simulink model "task2_2"  (R2023a)
settings: Solver=VariableStepAuto  StartTime=0.0  StopTime=10.0  RelTol=1e-3
settings Model: Creator=vasil  LastModifiedBy=vasil

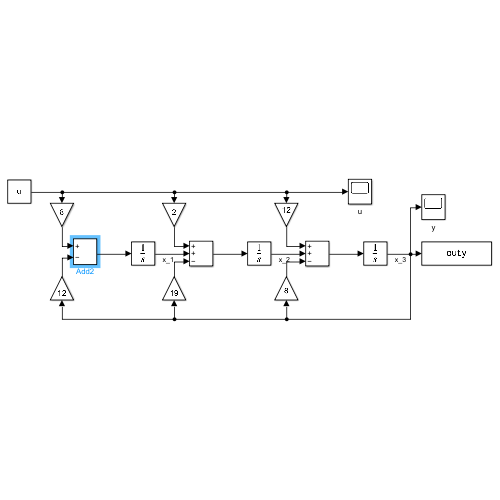
[thumbnail: Simulink's stored preview of the top-level diagram]
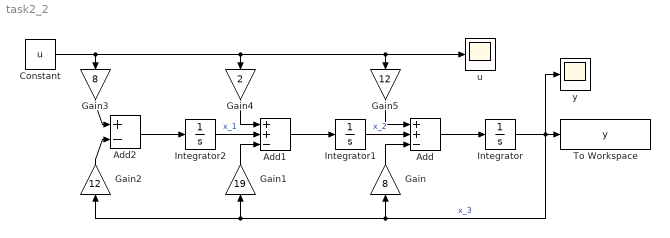
== system task2_2 ==
  Add : Sum  Inputs=++-
  Add1 : Sum  Inputs=++-
  Add2 : Sum  Inputs=+-
  Constant : Constant  Value=u
  Gain : Gain  Gain=8
  Gain1 : Gain  Gain=19
  Gain2 : Gain  Gain=12
  Gain3 : Gain  Gain=8
  Gain4 : Gain  Gain=2
  Gain5 : Gain  Gain=12
  Integrator : Integrator
  Integrator1 : Integrator
  Integrator2 : Integrator
  To Workspace : ToWorkspace  VariableName=y  SaveFormat=Timeseries  SampleTime=-1
  u : Scope
  y : Scope
  wires:
  Integrator/1 -> y/1, To Workspace/1, Gain2/1, Gain1/1, Gain/1  "x_3"
  Add/1 -> Integrator/1
  Integrator1/1 -> Add/2  "x_2"
  Add1/1 -> Integrator1/1
  Gain1/1 -> Add1/3
  Gain/1 -> Add/3
  Gain2/1 -> Add2/2
  Integrator2/1 -> Add1/2  "x_1"
  Add2/1 -> Integrator2/1
  Gain3/1 -> Add2/1
  Constant/1 -> Gain4/1, u/1, Gain5/1, Gain3/1
  Gain4/1 -> Add1/1
  Gain5/1 -> Add/1
